simulink library "TMCI_lib"  (Simulink 7.5)
settings: Solver=ode45  StartTime=0.0  StopTime=10.0  RelTol=1e-3
values from neighbouring files (symbols this model uses):
  p_TMCI_TMTemp_degC = Simulink.Parameter    [TMCI_par.m]
  p_TMCI_TMTempEnbl_bool = Simulink.Parameter    [TMCI_par.m]
undefined symbols (not defined in the file or in its folder): p_bool_False_M, p_bool_True_M, p_single_Zero_M
libraries: BaseOperationLib_Browser x7, PES_CZ_FAW x2, simulink x1
settings Model: Creator=wuaibin  LastModifiedBy=wuaibin

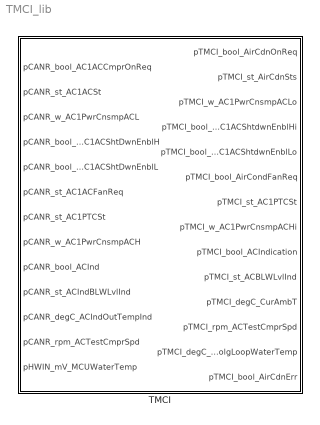
== system TMCI_lib ==
  TMCI : Subsystem  TreatAsAtomicUnit=on

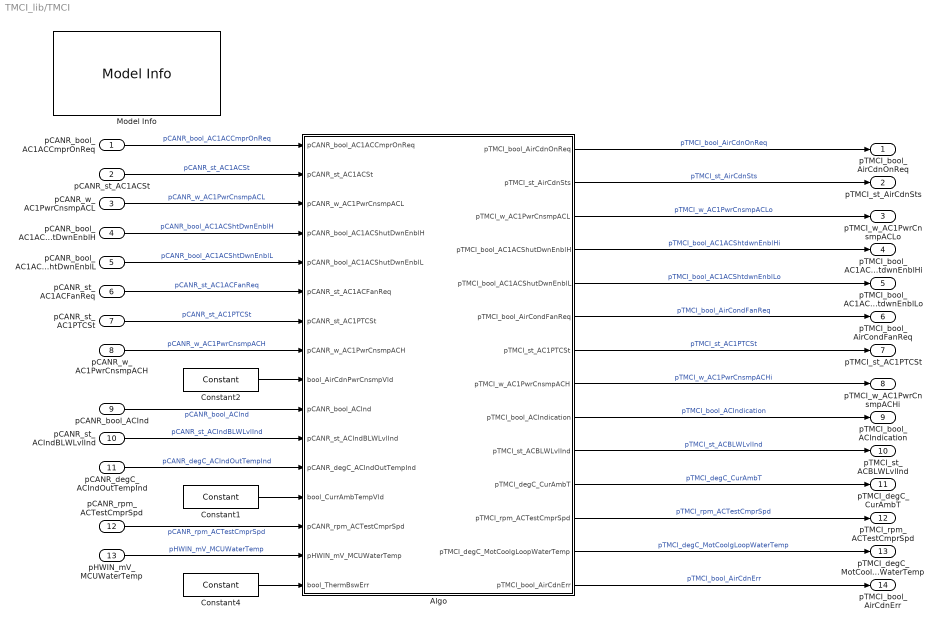
== system TMCI_lib/TMCI ==
  pCANR_bool_AC1ACCmprOnReq : Inport  OutDataType=fixdt(1, 16)  OutScaling=2^0
  pCANR_st_AC1ACSt : Inport  Port=2  OutDataType=fixdt(1, 16)  OutScaling=2^0
  pCANR_w_AC1PwrCnsmpACL : Inport  Port=3  OutDataType=fixdt(1, 16)  OutScaling=2^0
  pCANR_bool_AC1ACShtDwnEnblH : Inport  Port=4  OutDataType=fixdt(1, 16)  OutScaling=2^0
  pCANR_bool_AC1ACShtDwnEnblL : Inport  Port=5  OutDataType=fixdt(1, 16)  OutScaling=2^0
  pCANR_st_AC1ACFanReq : Inport  Port=6  OutDataType=fixdt(1, 16)  OutScaling=2^0
  pCANR_st_AC1PTCSt : Inport  Port=7  OutDataType=fixdt(1, 16)  OutScaling=2^0
  pCANR_w_AC1PwrCnsmpACH : Inport  Port=8  OutDataType=fixdt(1, 16)  OutScaling=2^0
  pCANR_bool_ACInd : Inport  Port=9  OutDataType=fixdt(1, 16)  OutScaling=2^0
  pCANR_st_ACIndBLWLvlInd : Inport  Port=10  OutDataType=fixdt(1, 16)  OutScaling=2^0
  pCANR_degC_ACIndOutTempInd : Inport  Port=11  OutDataType=fixdt(1, 16)  OutScaling=2^0
  pCANR_rpm_ACTestCmprSpd : Inport  Port=12  OutDataType=fixdt(1, 16)  OutScaling=2^0
  pHWIN_mV_MCUWaterTemp : Inport  Port=13  OutDataType=fixdt(1, 16)  OutScaling=2^0
  Algo : Subsystem
  Constant1 : BaseOperationLib_Browser/Sources&Sinks/Constant  Value=p_bool_True_M  OutMin=[]  OutMax=[]  OutDataType=fixdt(1, 16)  ConRadixGroup=Use specified scaling  OutScaling=2^0  OutDataTypeStr=Inherit: Inherit from 'Constant value'
  Constant2 : BaseOperationLib_Browser/Sources&Sinks/Constant  Value=p_bool_True_M  OutMin=[]  OutMax=[]  OutDataType=fixdt(1, 16)  ConRadixGroup=Use specified scaling  OutScaling=2^0  OutDataTypeStr=Inherit: Inherit from 'Constant value'
  Constant4 : BaseOperationLib_Browser/Sources&Sinks/Constant  Value=p_bool_False_M  OutMin=[]  OutMax=[]  OutDataTypeMode=uint32  OutDataType=fixdt(1, 16)  ConRadixGroup=Use specified scaling  OutScaling=2^0  OutDataTypeStr=uint32
  Model Info : simulink/Model-Wide Utilities/Model Info  SystemSampleTime=-1  InitialBlockCM=None  BlockCM=None  Frame=on  DisplayStringWithTags=Model Info\nCreated: %<Created>\nCreator: zhangqiang  HorizontalTextAlignment=Center  LeftAlignmentValue=0.5  SourceBlockDiagram=HQEV_HCU  TagMaxNumber=20
  pTMCI_bool_AirCdnOnReq : Outport  OutDataType=fixdt(1, 16)  OutScaling=2^0
  pTMCI_st_AirCdnSts : Outport  Port=2  OutDataType=fixdt(1, 16)  OutScaling=2^0
  pTMCI_w_AC1PwrCnsmpACLo : Outport  Port=3  OutDataType=fixdt(1, 16)  OutScaling=2^0
  pTMCI_bool_AC1ACShtdwnEnblHi : Outport  Port=4  OutDataType=fixdt(1, 16)  OutScaling=2^0
  pTMCI_bool_AC1ACShtdwnEnblLo : Outport  Port=5  OutDataType=fixdt(1, 16)  OutScaling=2^0
  pTMCI_bool_AirCondFanReq : Outport  Port=6  OutDataType=fixdt(1, 16)  OutScaling=2^0
  pTMCI_st_AC1PTCSt : Outport  Port=7  OutDataType=fixdt(1, 16)  OutScaling=2^0
  pTMCI_w_AC1PwrCnsmpACHi : Outport  Port=8  OutDataType=fixdt(1, 16)  OutScaling=2^0
  pTMCI_bool_ACIndication : Outport  Port=9  OutDataType=fixdt(1, 16)  OutScaling=2^0
  pTMCI_st_ACBLWLvlInd : Outport  Port=10  OutDataType=fixdt(1, 16)  OutScaling=2^0
  pTMCI_degC_CurAmbT : Outport  Port=11  OutDataType=fixdt(1, 16)  OutScaling=2^0
  pTMCI_rpm_ACTestCmprSpd : Outport  Port=12  OutDataType=fixdt(1, 16)  OutScaling=2^0
  pTMCI_degC_MotCoolgLoopWaterTemp : Outport  Port=13  OutDataType=fixdt(1, 16)  OutScaling=2^0
  pTMCI_bool_AirCdnErr : Outport  Port=14  OutDataType=fixdt(1, 16)  OutScaling=2^0
  wires:
  pCANR_w_AC1PwrCnsmpACH/1 -> Algo/8(pCANR_w_AC1PwrCnsmpACH)  "pCANR_w_AC1PwrCnsmpACH"
  pCANR_w_AC1PwrCnsmpACL/1 -> Algo/3(pCANR_w_AC1PwrCnsmpACL)  "pCANR_w_AC1PwrCnsmpACL"
  Algo/14(pTMCI_bool_AirCdnErr) -> pTMCI_bool_AirCdnErr/1  "pTMCI_bool_AirCdnErr"
  Algo/1(pTMCI_bool_AirCdnOnReq) -> pTMCI_bool_AirCdnOnReq/1  "pTMCI_bool_AirCdnOnReq"
  pCANR_bool_AC1ACCmprOnReq/1 -> Algo/1(pCANR_bool_AC1ACCmprOnReq)  "pCANR_bool_AC1ACCmprOnReq"
  pCANR_st_AC1ACSt/1 -> Algo/2(pCANR_st_AC1ACSt)  "pCANR_st_AC1ACSt"
  pCANR_degC_ACIndOutTempInd/1 -> Algo/12(pCANR_degC_ACIndOutTempInd)  "pCANR_degC_ACIndOutTempInd"
  Algo/2(pTMCI_st_AirCdnSts) -> pTMCI_st_AirCdnSts/1  "pTMCI_st_AirCdnSts"
  Algo/6(pTMCI_bool_AirCondFanReq) -> pTMCI_bool_AirCondFanReq/1  "pTMCI_bool_AirCondFanReq"
  pCANR_st_AC1ACFanReq/1 -> Algo/6(pCANR_st_AC1ACFanReq)  "pCANR_st_AC1ACFanReq"
  Algo/13(pTMCI_degC_MotCoolgLoopWaterTemp) -> pTMCI_degC_MotCoolgLoopWaterTemp/1  "pTMCI_degC_MotCoolgLoopWaterTemp"
  pHWIN_mV_MCUWaterTemp/1 -> Algo/15(pHWIN_mV_MCUWaterTemp)  "pHWIN_mV_MCUWaterTemp"
  pCANR_bool_AC1ACShtDwnEnblH/1 -> Algo/4(pCANR_bool_AC1ACShutDwnEnblH)  "pCANR_bool_AC1ACShtDwnEnblH"
  pCANR_bool_AC1ACShtDwnEnblL/1 -> Algo/5(pCANR_bool_AC1ACShutDwnEnblL)  "pCANR_bool_AC1ACShtDwnEnblL"
  pCANR_st_AC1PTCSt/1 -> Algo/7(pCANR_st_AC1PTCSt)  "pCANR_st_AC1PTCSt"
  Algo/4(pTMCI_bool_AC1ACShutDwnEnblH) -> pTMCI_bool_AC1ACShtdwnEnblHi/1  "pTMCI_bool_AC1ACShtdwnEnblHi"
  Algo/5(pTMCI_bool_AC1ACShutDwnEnblL) -> pTMCI_bool_AC1ACShtdwnEnblLo/1  "pTMCI_bool_AC1ACShtdwnEnblLo"
  Algo/9(pTMCI_bool_ACIndication) -> pTMCI_bool_ACIndication/1  "pTMCI_bool_ACIndication"
  Algo/10(pTMCI_st_ACBLWLvlInd) -> pTMCI_st_ACBLWLvlInd/1  "pTMCI_st_ACBLWLvlInd"
  pCANR_bool_ACInd/1 -> Algo/10(pCANR_bool_ACInd)  "pCANR_bool_ACInd"
  pCANR_st_ACIndBLWLvlInd/1 -> Algo/11(pCANR_st_ACIndBLWLvlInd)  "pCANR_st_ACIndBLWLvlInd"
  pCANR_rpm_ACTestCmprSpd/1 -> Algo/14(pCANR_rpm_ACTestCmprSpd)  "pCANR_rpm_ACTestCmprSpd"
  Algo/7(pTMCI_st_AC1PTCSt) -> pTMCI_st_AC1PTCSt/1  "pTMCI_st_AC1PTCSt"
  Algo/11(pTMCI_degC_CurAmbT) -> pTMCI_degC_CurAmbT/1  "pTMCI_degC_CurAmbT"
  Algo/12(pTMCI_rpm_ACTestCmprSpd) -> pTMCI_rpm_ACTestCmprSpd/1  "pTMCI_rpm_ACTestCmprSpd"
  Algo/3(pTMCI_w_AC1PwrCnsmpACL) -> pTMCI_w_AC1PwrCnsmpACLo/1  "pTMCI_w_AC1PwrCnsmpACLo"
  Algo/8(pTMCI_w_AC1PwrCnsmpACH) -> pTMCI_w_AC1PwrCnsmpACHi/1  "pTMCI_w_AC1PwrCnsmpACHi"
  Constant4/1 -> Algo/16(bool_ThermBswErr)
  Constant1/1 -> Algo/13(bool_CurrAmbTempVld)
  Constant2/1 -> Algo/9(bool_AirCdnPwrCnsmpVld)

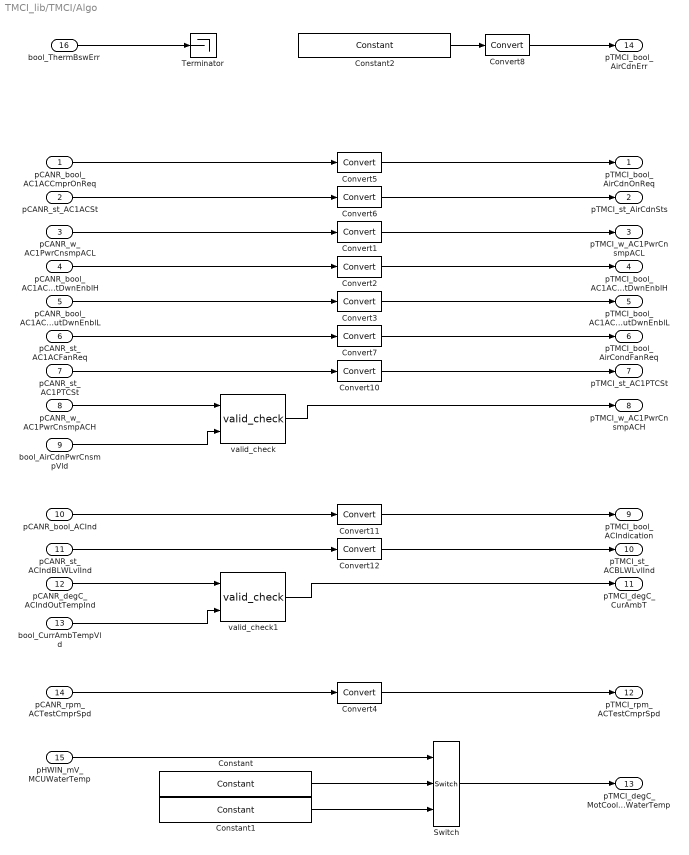
== system TMCI_lib/TMCI/Algo ==
  pCANR_bool_AC1ACCmprOnReq : Inport  OutDataType=fixdt(1, 16)  OutScaling=2^0
  pCANR_st_AC1ACSt : Inport  Port=2  OutDataType=fixdt(1, 16)  OutScaling=2^0
  pCANR_w_AC1PwrCnsmpACL : Inport  Port=3  OutDataType=fixdt(1, 16)  OutScaling=2^0
  pCANR_bool_AC1ACShutDwnEnblH : Inport  Port=4  OutDataType=fixdt(1, 16)  OutScaling=2^0
  pCANR_bool_AC1ACShutDwnEnblL : Inport  Port=5  OutDataType=fixdt(1, 16)  OutScaling=2^0
  pCANR_st_AC1ACFanReq : Inport  Port=6  OutDataType=fixdt(1, 16)  OutScaling=2^0
  pCANR_st_AC1PTCSt : Inport  Port=7  OutDataType=fixdt(1, 16)  OutScaling=2^0
  pCANR_w_AC1PwrCnsmpACH : Inport  Port=8  OutDataType=fixdt(1, 16)  OutScaling=2^0
  bool_AirCdnPwrCnsmpVld : Inport  Port=9  OutDataType=fixdt(1, 16)  OutScaling=2^0
  pCANR_bool_ACInd : Inport  Port=10  OutDataType=fixdt(1, 16)  OutScaling=2^0
  pCANR_st_ACIndBLWLvlInd : Inport  Port=11  OutDataType=fixdt(1, 16)  OutScaling=2^0
  pCANR_degC_ACIndOutTempInd : Inport  Port=12  OutDataType=fixdt(1, 16)  OutScaling=2^0
  bool_CurrAmbTempVld : Inport  Port=13  OutDataType=fixdt(1, 16)  OutScaling=2^0
  pCANR_rpm_ACTestCmprSpd : Inport  Port=14  OutDataType=fixdt(1, 16)  OutScaling=2^0
  pHWIN_mV_MCUWaterTemp : Inport  Port=15  OutDataType=fixdt(1, 16)  OutScaling=2^0
  bool_ThermBswErr : Inport  Port=16  OutDataType=fixdt(1, 16)  OutScaling=2^0
  Constant : BaseOperationLib_Browser/Sources&Sinks/Constant  Value=p_TMCI_TMTempEnbl_bool  OutMin=[]  OutMax=[]  OutDataType=fixdt(1, 16)  ConRadixGroup=Use specified scaling  OutScaling=2^0  OutDataTypeStr=Inherit: Inherit from 'Constant value'
  Constant1 : BaseOperationLib_Browser/Sources&Sinks/Constant  Value=p_TMCI_TMTemp_degC  OutMin=[]  OutMax=[]  OutDataType=fixdt(1, 16)  ConRadixGroup=Use specified scaling  OutScaling=2^0  OutDataTypeStr=Inherit: Inherit from 'Constant value'
  Constant2 : BaseOperationLib_Browser/Sources&Sinks/Constant  Value=p_single_Zero_M  OutMin=[]  OutMax=[]  OutDataType=fixdt(1, 16)  ConRadixGroup=Use specified scaling  OutScaling=2^0  OutDataTypeStr=Inherit: Inherit from 'Constant value'
  Convert{1..8,10..12} (11 alike) : DataTypeConversion  OutDataType=fixdt(1, 16)  OutScaling=2^0
  Switch : BaseOperationLib_Browser/Signal Routing Changed/Switch  Criteria=u2 ~= 0  Threshold=1  InputSameDT=on  OutMin=[]  OutMax=[]  OutDataType=fixdt(1,16,0)  OutScaling=[]  SaturateOnIntegerOverflow=on
  Terminator : Terminator
  valid_check : PES_CZ_FAW/Discontinuities/valid_check  SystemSampleTime=-1  init=0
  valid_check1 : PES_CZ_FAW/Discontinuities/valid_check  SystemSampleTime=-1  init=0
  pTMCI_bool_AirCdnOnReq : Outport  OutDataType=fixdt(1, 16)  OutScaling=2^0
  pTMCI_st_AirCdnSts : Outport  Port=2  OutDataType=fixdt(1, 16)  OutScaling=2^0
  pTMCI_w_AC1PwrCnsmpACL : Outport  Port=3  OutDataType=fixdt(1, 16)  OutScaling=2^0
  pTMCI_bool_AC1ACShutDwnEnblH : Outport  Port=4  OutDataType=fixdt(1, 16)  OutScaling=2^0
  pTMCI_bool_AC1ACShutDwnEnblL : Outport  Port=5  OutDataType=fixdt(1, 16)  OutScaling=2^0
  pTMCI_bool_AirCondFanReq : Outport  Port=6  OutDataType=fixdt(1, 16)  OutScaling=2^0
  pTMCI_st_AC1PTCSt : Outport  Port=7  OutDataType=fixdt(1, 16)  OutScaling=2^0
  pTMCI_w_AC1PwrCnsmpACH : Outport  Port=8  OutDataType=fixdt(1, 16)  OutScaling=2^0
  pTMCI_bool_ACIndication : Outport  Port=9  OutDataType=fixdt(1, 16)  OutScaling=2^0
  pTMCI_st_ACBLWLvlInd : Outport  Port=10  OutDataType=fixdt(1, 16)  OutScaling=2^0
  pTMCI_degC_CurAmbT : Outport  Port=11  OutDataType=fixdt(1, 16)  OutScaling=2^0
  pTMCI_rpm_ACTestCmprSpd : Outport  Port=12  OutDataType=fixdt(1, 16)  OutScaling=2^0
  pTMCI_degC_MotCoolgLoopWaterTemp : Outport  Port=13  OutDataType=fixdt(1, 16)  OutScaling=2^0
  pTMCI_bool_AirCdnErr : Outport  Port=14  OutDataType=fixdt(1, 16)  OutScaling=2^0
  wires:
  pCANR_w_AC1PwrCnsmpACH/1 -> valid_check/1
  bool_ThermBswErr/1 -> Terminator/1
  pCANR_bool_AC1ACCmprOnReq/1 -> Convert5/1
  pCANR_st_AC1ACSt/1 -> Convert6/1
  pCANR_st_AC1ACFanReq/1 -> Convert7/1
  bool_AirCdnPwrCnsmpVld/1 -> valid_check/2
  pHWIN_mV_MCUWaterTemp/1 -> Switch/1
  Switch/1 -> pTMCI_degC_MotCoolgLoopWaterTemp/1
  Constant/1 -> Switch/2
  Constant1/1 -> Switch/3
  pCANR_w_AC1PwrCnsmpACL/1 -> Convert1/1
  pCANR_bool_AC1ACShutDwnEnblH/1 -> Convert2/1
  pCANR_bool_AC1ACShutDwnEnblL/1 -> Convert3/1
  Convert1/1 -> pTMCI_w_AC1PwrCnsmpACL/1
  Convert2/1 -> pTMCI_bool_AC1ACShutDwnEnblH/1
  Convert3/1 -> pTMCI_bool_AC1ACShutDwnEnblL/1
  Convert5/1 -> pTMCI_bool_AirCdnOnReq/1
  Convert6/1 -> pTMCI_st_AirCdnSts/1
  Convert7/1 -> pTMCI_bool_AirCondFanReq/1
  pCANR_st_AC1PTCSt/1 -> Convert10/1
  Convert10/1 -> pTMCI_st_AC1PTCSt/1
  bool_CurrAmbTempVld/1 -> valid_check1/2
  Convert11/1 -> pTMCI_bool_ACIndication/1
  pCANR_bool_ACInd/1 -> Convert11/1
  Convert12/1 -> pTMCI_st_ACBLWLvlInd/1
  pCANR_st_ACIndBLWLvlInd/1 -> Convert12/1
  valid_check/1 -> pTMCI_w_AC1PwrCnsmpACH/1
  valid_check1/1 -> pTMCI_degC_CurAmbT/1
  pCANR_degC_ACIndOutTempInd/1 -> valid_check1/1
  pCANR_rpm_ACTestCmprSpd/1 -> Convert4/1
  Convert4/1 -> pTMCI_rpm_ACTestCmprSpd/1
  Constant2/1 -> Convert8/1
  Convert8/1 -> pTMCI_bool_AirCdnErr/1
